simulink model "Fig53"  (R2014b)
settings: Solver=ode3  StartTime=0.0  StopTime=.05  FixedStep=1e-3  RelTol=1e-3
libraries: commrandsrc2 x3, commutil2 x1
settings Model: Creator=Silage  LastModifiedBy=Silage

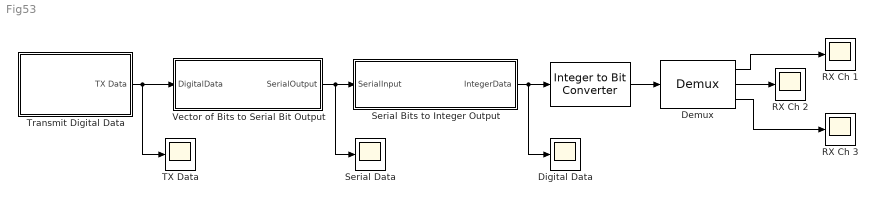
== system Fig53 ==
  " " : commutil2/Integer to Bit Converter  nbits=3  signedInputValues=Unsigned  bitOrder=LSB first  outDtype=Inherit via internal rule
  Demux : Demux  Outputs=3
  Digital Data : Scope
      settings: SaveName=ScopeData6
  RX Ch 1 : Scope
  RX Ch 2 : Scope
  RX Ch 3 : Scope
      settings: SaveName=ScopeData8
  Serial Bits to Integer Output : MATLAB Function  TreatAsAtomicUnit=on
  Serial Data : Scope
      settings: SaveName=ScopeData3
  TX Data : Scope
      settings: SaveName=ScopeData2
  Transmit Digital Data : Subsystem
  Vector of Bits to Serial Bit Output : MATLAB Function  TreatAsAtomicUnit=on
  wires:
  Demux/1 -> RX Ch 1/1
  Demux/2 -> RX Ch 2/1
  Vector of Bits to Serial Bit Output/1(SerialOutput) -> Serial Bits to Integer Output/1(SerialInput), Serial Data/1
  Serial Bits to Integer Output/1(IntegerData) -> " "/1, Digital Data/1
  " "/1 -> Demux/1
  Transmit Digital Data/1(TX Data) -> Vector of Bits to Serial Bit Output/1(DigitalData), TX Data/1
  Demux/3 -> RX Ch 3/1

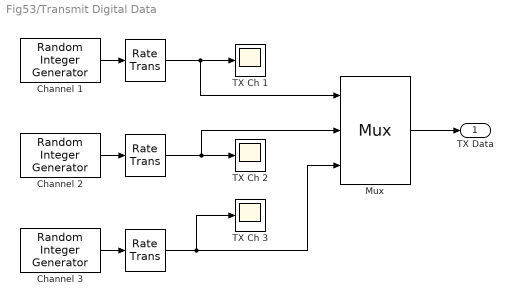
== system Fig53/Transmit Digital Data ==
  " " : RateTransition  OutPortSampleTime=1e-3
  "  " : RateTransition  OutPortSampleTime=1e-3
  "    " : RateTransition  OutPortSampleTime=1e-3
  Channel 1 : commrandsrc2/Random Integer Generator  mul=2  seed=37  Ts=4e-3  frameBased=off  sampPerFrame=1  orient=on  outDataType=double
  Channel 2 : commrandsrc2/Random Integer Generator  mul=2  seed=59  Ts=4e-3  frameBased=off  sampPerFrame=1  orient=on  outDataType=double
  Channel 3 : commrandsrc2/Random Integer Generator  mul=2  seed=42  Ts=2e-3  frameBased=off  sampPerFrame=1  orient=on  outDataType=double
  Mux : Mux  Inputs=3
      settings: DisplayOption=signals
  TX Ch 1 : Scope
      settings: SaveName=ScopeData4
  TX Ch 2 : Scope
      settings: SaveName=ScopeData5
  TX Ch 3 : Scope
      settings: SaveName=ScopeData7
  TX Data : Outport
  wires:
  Mux/1 -> TX Data/1
  Channel 1/1 -> " "/1
  " "/1 -> Mux/1, TX Ch 1/1
  Channel 2/1 -> "  "/1
  "  "/1 -> Mux/2, TX Ch 2/1
  Channel 3/1 -> "    "/1
  "    "/1 -> TX Ch 3/1, Mux/3

== matlab function Fig53/Serial Bits to Integer Output ==
  data: SerialInput input; IntegerData output
function IntegerData = fcn(SerialInput)
%#codegen

persistent SmpDat  SmpNum SmpDatOld

if isempty(SmpNum)
    SmpNum = 0;
    SmpDat = 0;
    SmpDatOld = 0;
    IntegerData = 0; %#ok<*NASGU>
end

SmpNum = SmpNum + 1;
ID = 0;
if (SmpNum == 1)
    SmpDat = SerialInput;
end
if (SmpNum == 2)
    SmpDat = SmpDat + 2*SerialInput;
    SmpDatOld = SmpDat;
end
if (SmpNum == 3)
    ID = SmpDat + 4*SerialInput; 
end
if (SmpNum == 4)
    ID = SmpDatOld + 4*SerialInput;
    SmpNum =0;
end
IntegerData = ID;

end

== matlab function Fig53/Vector of Bits to Serial Bit Output ==
  data: DigitalData input; SerialOutput output
function SerialOutput = fcn(DigitalData)
%#codegen
persistent SmpDat SmpNum SmpCh3

if isempty(SmpNum)
    SmpNum = 0;
    SmpDat = DigitalData; %#ok<NASGU>
    SmpCh3 = 0;
    SerialOutput = 0; %#ok<NASGU>
end

SmpNum = SmpNum + 1;
SO = 0;
SmpDat = DigitalData;
if (SmpNum == 1)
    SO = SmpDat(1);
end
if (SmpNum == 2)
    SO = SmpDat(2);
    SmpCh3 = SmpDat(3);
end
if (SmpNum == 3)
    SO = SmpCh3;
    SmpCh3 = SmpDat(3);
end
if (SmpNum ==4)
    SO = SmpCh3;
    SmpNum = 0;
end
SerialOutput = SO;

end
